simulink model "modelo_2"  (R2020a)
settings: Solver=VariableStepAuto  StartTime=0.0  StopTime=180  RelTol=1e-3
values from neighbouring files (symbols this model uses):
  Pnom = 2e6    (= 2000000)    [Parametros.m]
  Pnom1 = 2e6    (= 2000000)    [Parametros.m]
libraries: powerlib x7, re_lib x2, powerlib_meascontrol x1
settings Model: Creator=octad  LastModifiedBy=octad

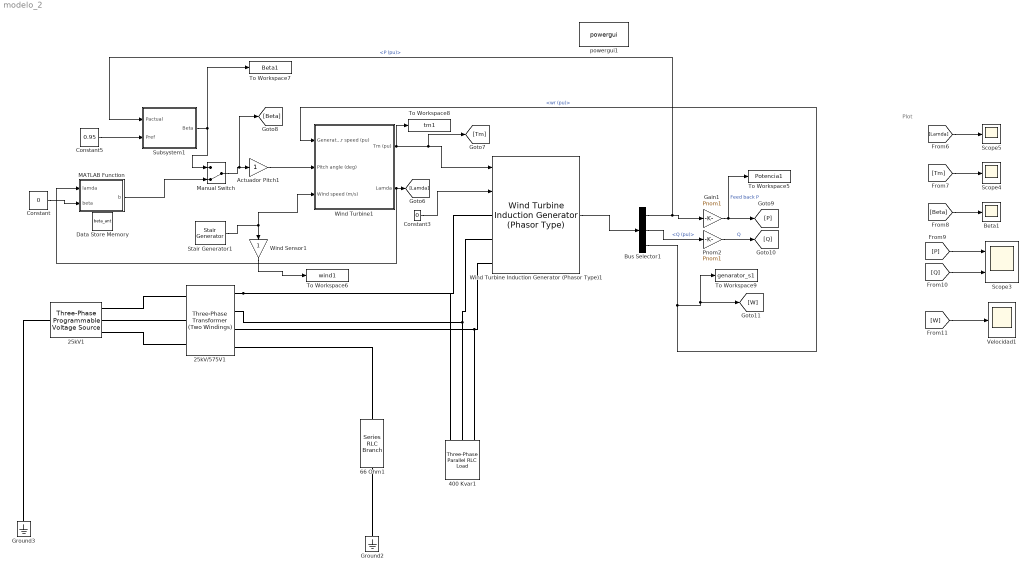
== system modelo_2 ==
  note: Plot
  25kV/575V1 : powerlib/Elements/Three-Phase Transformer (Two Windings)  Winding1Connection=Yg  Winding2Connection=Yn  CoreType=Three single-phase transformers  SetSaturation=off  Hysteresis=off  DataFile='hysteresis'  SetInitialFlux=off  Measurements=None  UNITS=pu  NominalPower=[ 4e6 , 60 ]  Winding1=[ 25e3 , 0.025/30 , 0.025]  Winding2=[575 , 0.025/30 , 0.025 ]  Rm=500  Lm=inf  L0=0.5  Saturation=[ 0,0 ; 0.0024,1.2 ; 1.0,1.52 ]  InitialFluxes=[ 0.8 , -0.8 , 0.7 ]  BreakLoop=off  DiscreteSolver=Trapezoidal iterative  DataType=off  TransfoNumber=1
  25kV1 : powerlib/Electrical Sources/Three-Phase Programmable Voltage Source  PositiveSequence="[25000  0 60]"  VariationEntity=None  VariationType=Table of time-amplitude pairs  VariationTypeAlt=Step  VariationStep=0.5  VariationRate=10  VariationMagnitude=0.3  VariationFrequency=2  VariationTiming=[1 2]  VariationPhaseA=off  Amplitudes=[1 0.8 1.2 1.0]  TimeValues=[0 0.1 0.15 0.2]  HarmonicGeneration=off  HarmonicA=[3 0.2 -25 0]  HarmonicB=[2 0.15 35 2]  Timing="[0.05  3]"  BusType=swing  Pref=0  Qref=0  Qmin=-inf  Qmax=inf
  400 Kvar1 : powerlib/Elements/Three-Phase Parallel RLC Load  LConnTagsString=A|B|C  Configuration=Delta  NominalVoltage=575  Vabc=[1e3 1e3 1e3]  Vabcp=[1e3 1e3 1e3]  NominalFrequency=60  UnbalancedPower=off  ActivePower=0  InductivePower=0  CapacitivePower=400e3  Pabc=[10e3 9e3 11e3]  QLabc=[100 90 110]  QCabc=[100 90 110]  Pabcp=[10e3 9e3 11e3]  QLabcp=[100 90 110]  QCabcp=[100 90 110]  Measurements=None  LoadType=constant Z
  66 Ohm1 : powerlib/Elements/Series RLC Branch  LConnTagsString=__new0  RConnTagsString=__new0  BranchType=R  Resistance=66  Inductance=1e-3  SetiL0=off  InitialCurrent=0  Capacitance=1e-6  Setx0=off  InitialVoltage=0  Measurements=None
  Actuador Pitch1 : Gain
  Beta1 : Scope
  Bus Selector1 : BusSelector  OutputSignals=P (pu),Q (pu),wr (pu)
  Constant : Constant  Value=0
  Constant3 : Constant  Value=0
  Constant5 : Constant  Value=0.95
  Data Store Memory : DataStoreMemory  DataStoreName=beta_ant  ReadBeforeWriteMsg=warning  WriteAfterWriteMsg=warning  WriteAfterReadMsg=warning  ShowAdditionalParam=off  OutDataTypeStr=double
  Gain1 : Gain  Gain=Pnom1
  Ground2 : powerlib/Elements/Ground  LConnTagsString=a
  Ground3 : powerlib/Elements/Ground  LConnTagsString=a
  MATLAB Function : MATLAB Function  TreatAsAtomicUnit=on
  Manual Switch : ManualSwitch  CurrentSetting=0
  Pnom2 : Gain  Gain=Pnom1
  Scope3 : Scope  NumInputPorts=2
  Scope4 : Scope
  Scope5 : Scope
  Stair Generator1 : powerlib_meascontrol/Pulse & Signal Generators/Stair Generator  t=[0, 10, 20, 30, 40, 60,70,90]  e=[3, 7, 11, 13, 18, 13,11,12]  Ts=0
  Subsystem1 : Subsystem
  To Workspace5 : ToWorkspace  VariableName=Potencia1  SaveFormat=Timeseries  SampleTime=-1
  To Workspace6 : ToWorkspace  VariableName=wind1  SaveFormat=Timeseries  SampleTime=-1
  To Workspace7 : ToWorkspace  VariableName=Beta1  SaveFormat=Timeseries  SampleTime=-1
  To Workspace8 : ToWorkspace  VariableName=tm1  SaveFormat=Timeseries  SampleTime=-1
  To Workspace9 : ToWorkspace  VariableName=genarator_s1  SaveFormat=Timeseries  SampleTime=-1
  Velocidad1 : Scope
  Wind Sensor1 : Gain
  Wind Turbine Induction Generator (Phasor Type)1 : re_lib/Wind Generation/Wind Turbine Induction Generator (Phasor Type)  ExternalTm=on  nom=[Pnom1/0.9, 575, 60]  sta=[ 0.004843, 0.1248]  rot=[ 0.004377, 0.1791]  Lm=6.77  mec=[5.04, 0.01, 3]  init="[ -0.01,0,   0,0,0,   0,0,0 ]"  pitch_angle=0  Pmec=1.5e6  wind_base=12  speed_nom=1  P_wind_base=1  K_pitch_gain=[5 25]  pitch_max=45  pitch_rate=2
      settings: SourceProductBaseCode=PS
  Wind Turbine1 : Subsystem  AncestorBlock=re_lib/Wind Generation/Wind Turbine  DialogController=POWERSYS.PowerSysDialog  mask(Wind Turbine){Pnom=Pnom, Pelec_base=Pnom1/0.9, wind_base=12, P_wind_base=0.5, speed_nom=1, pitch_angle=0, c1_c6=[0.51763          116          0.4            5           21     0.006795], cp_nom=0.48, lambda_nom=8.1}
      mask prompts: Pnom "Nominal mechanical output power (W):"; Pelec_base "Base power of the electrical generator (VA):"; wind_base "Base wind speed (m/s):"; P_wind_base "Maximum power at base wind speed (pu of nominal mechanical power):"; speed_nom "Base rotational speed (p.u. of base generator speed):"; pitch_angle "Pitch angle beta to display wind-turbine power characteristics (beta >=0)  (deg):"
      mask help:
      | This block implements a variable pitch wind turbine model. The performance coefficient Cp of the turbine is the mechanical output power of the turbine divided by wind power and a function of wind speed, rotational speed, and pitch angle (beta). Cp reaches its maximum value at zero beta. Select the wind-turbine power characteristics display to plot the turbine characteristics at the specified pitch angle.
      |
      | The first input is the generator speed in per unit of the generator base speed. For a synchronous or asynchronous generator, the base speed is the synchronous speed. For a permanent-magnet generator, the base speed is defined as the speed producing nominal voltage at  no load. The second input is the blade pitch angle (beta) in degrees. The third input is the wind speed in m/s.
      |
      | The output is the torque applied to the generator shaft in per unit of the generator ratings.
      |
      | The turbine inertia must be added to the generator inertia.
      mask init:
      | c1=c1_c6(1);c2=c1_c6(2);c3=c1_c6(3);c4=c1_c6(4);c5=c1_c6(5);c6=c1_c6(6);
      | 
      | if Pnom<=0
      |     error(message('physmod:powersys:common:GreaterThan',getfullname(gcbh),'Nominal mechanical output power',0));
      | end
      | if Pelec_base<=0
      |     error(message('physmod:powersys:common:GreaterThan',getfullname(gcbh),'Base power of the electrical generator',0));
      | end
      | if wind_base<=0
      |     error(message('physmod:powersys:common:GreaterThan',getfullname(gcbh),'Base wind speed (m/s)',0));
      | end
      | if P_wind_base<=0
      |     error(message('physmod:powersys:common:GreaterThan',getfullname(gcbh),'Maximum power at base wind speed',0));
      | end
      | power_initmask();
      settings: OpenFcn=sps_rtmsupport('OpenFcn',gcbh)
      mask Help: helpview(psbhelp);
      mask DialogControl DisplayTurbChar Prompt: Display wind turbine power characteristics
      mask DialogControl DisplayTurbChar Callback: WindTurbinePlot(gcb)
      mask Display: disp('');
  powergui1 : powerlib/powergui  Priority=1  SimulationMode=Phasor  SampleTime=50e-6  frequency=60  Iterations=50  frequencyindice=60  Pbase=100e6  ErrMax=1e-4  UnitsV=kV  UnitsW=MW  buscounter=0  FunctionMessages=off  echomessages=off  EnableUseOfTLC=off  CurrentSourceSwitches=off  DisableSnubberDevices=off  DisableRonSwitches=off  DisableVfSwitches=off  DisplayEquations=off  AutomaticDiscreteSolvers=off  SolverType=Tustin/Backward Euler (TBE)  Interpol=off  ExternalGateDelay=off  methode=off  Ts=100  x0status=blocks  SPID=on  SwTol=0  HookPort=off  NonlinearTolerance=1e-4  nMaxIteration=100  ContinueOnMaxIteration=off  RestoreLinks=warning  ResistiveCurrentMeasurement=off  Frange=[0:2:500]  Ylog=off  Xlog=on  ShowGrid=off  save=off  variable=ZData  structure=0  ZoomFFT=off  StartTime=0.0  cycles=1  DisplayStyle=1  fundamental=60  FreqAxis=off  MaxFrequency=1000  frequencyindicesteady=1  RmsSteady=1  display=off
  wires:
  Actuador Pitch1/1 -> Wind Turbine1/2(Pitch angle (deg))
  Wind Sensor1/1 -> To Workspace6/1
  Wind Turbine1/2(Lamda) -> MATLAB Function/1(lamda), [Lamda]
  [P] -> Scope3/1
  Constant5/1 -> Subsystem1/2(Pref)
  Constant3/1 -> Wind Turbine Induction Generator (Phasor Type)1/2
  Wind Turbine Induction Generator (Phasor Type)1/1 -> Bus Selector1/1
  Bus Selector1/3 -> [W], To Workspace9/1, Wind Turbine1/1(Generator speed (pu))  "<wr (pu)>"
  Gain1/1 -> [P], To Workspace5/1  "Feed back P"
  Subsystem1/1(Beta) -> Manual Switch/1, To Workspace7/1
  Wind Turbine1/1(Tm (pu)) -> [Tm], Wind Turbine Induction Generator (Phasor Type)1/1, To Workspace8/1
  Bus Selector1/1 -> Subsystem1/1(Pactual), Gain1/1  "<P (pu)>"
  [W] -> Velocidad1/1
  Pnom2/1 -> [Q]  "Q"
  [Tm] -> Scope4/1
  Bus Selector1/2 -> Pnom2/1  "<Q (pu)>"
  [Beta] -> Beta1/1
  [Lamda] -> Scope5/1
  Stair Generator1/1 -> Wind Turbine1/3(Wind speed (m/s)), Wind Sensor1/1
  [Q] -> Scope3/2
  MATLAB Function/1(b) -> Manual Switch/2
  Manual Switch/1 -> [Beta], Actuador Pitch1/1
  Constant/1 -> MATLAB Function/2(beta)
  connections:
  25kV/575V1/RConn3 -- 400 Kvar1/LConn3 -- Wind Turbine Induction Generator (Phasor Type)1/LConn3
  25kV/575V1/RConn1 -- 400 Kvar1/LConn1 -- Wind Turbine Induction Generator (Phasor Type)1/LConn1
  25kV/575V1/RConn2 -- Wind Turbine Induction Generator (Phasor Type)1/LConn2 -- 400 Kvar1/LConn2
  25kV/575V1/RConn4 -- 66 Ohm1/LConn1
  Ground3/LConn1 -- 25kV1/LConn1
  25kV1/RConn3 -- 25kV/575V1/LConn3
  25kV1/RConn2 -- 25kV/575V1/LConn2
  25kV1/RConn1 -- 25kV/575V1/LConn1
  Ground2/LConn1 -- 66 Ohm1/RConn1

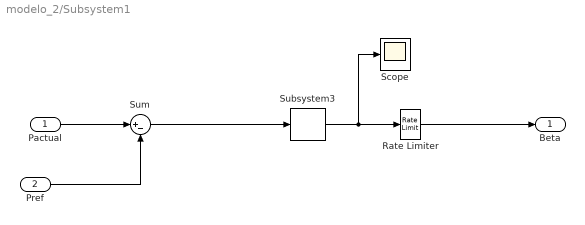
== system modelo_2/Subsystem1 ==
  Pactual : Inport
  Pref : Inport  Port=2
  "Rate Limiter   " : RateLimiter  RisingSlewLimit=2  FallingSlewLimit=-2
  Scope : Scope
  Subsystem3 : re_lib/Wind Generation/Wind Turbine Induction Generator (Phasor Type)/Subsystem3  Kp=5  Ki=25  Limits=[45 0]  Init=0
      settings: SourceProductBaseCode=PS
  Sum : Sum  Inputs=|+-
  Beta : Outport
  wires:
  Pref/1 -> Sum/2
  Subsystem3/1 -> Scope/1, "Rate Limiter   "/1
  "Rate Limiter   "/1 -> Beta/1
  Pactual/1 -> Sum/1
  Sum/1 -> Subsystem3/1

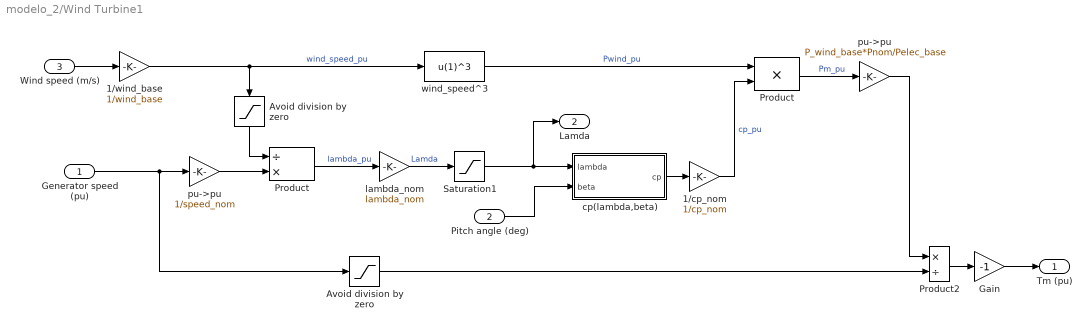
== system modelo_2/Wind Turbine1 ==
  Generator speed (pu) : Inport
  Pitch angle (deg) : Inport  Port=2
  Wind speed (m/s) : Inport  Port=3
  1/cp_nom : Gain  Gain=1/cp_nom  SaturateOnIntegerOverflow=on  OutDataTypeStr=Inherit: Same as input  ParamDataTypeStr=Inherit: Same as input
  1/wind_base : Gain  Gain=1/wind_base  SaturateOnIntegerOverflow=on  OutDataTypeStr=Inherit: Same as input  ParamDataTypeStr=Inherit: Same as input
  Avoid division by zero : Saturate  UpperLimit=1e6  LowerLimit=1e-6
  "Avoid division by zero " : Saturate  UpperLimit=inf  LowerLimit=1e-6
  Gain : Gain  Gain=-1  SaturateOnIntegerOverflow=on  OutDataTypeStr=Inherit: Same as input  ParamDataTypeStr=Inherit: Same as input
  Product : Product  Inputs=/*  SaturateOnIntegerOverflow=on  OutDataTypeStr=Inherit: Same as first input
  "Product " : Product  SaturateOnIntegerOverflow=on  OutDataTypeStr=Inherit: Same as first input
  Product2 : Product  Inputs=*/  InputSameDT=on  SaturateOnIntegerOverflow=on  OutDataTypeStr=Inherit: Same as first input
  Saturation1 : Saturate  UpperLimit=inf  LowerLimit=1e-6
  cp(lambda,beta) : Subsystem
  lambda_nom : Gain  Gain=lambda_nom  SaturateOnIntegerOverflow=on  OutDataTypeStr=Inherit: Same as input  ParamDataTypeStr=Inherit: Same as input
  pu->pu : Gain  Gain=P_wind_base*Pnom/Pelec_base  SaturateOnIntegerOverflow=on  OutDataTypeStr=Inherit: Same as input  ParamDataTypeStr=Inherit: Same as input
  "pu->pu " : Gain  Gain=1/speed_nom  SaturateOnIntegerOverflow=on  OutDataTypeStr=Inherit: Same as input  ParamDataTypeStr=Inherit: Same as input
  wind_speed^3 : Fcn  Expr=u(1)^3
  Tm (pu) : Outport  VectorParamsAs1DForOutWhenUnconnected=off
  Lamda : Outport  Port=2
  wires:
  Pitch angle (deg)/1 -> cp(lambda,beta)/2(beta)
  pu->pu/1 -> Product2/1
  cp(lambda,beta)/1(cp) -> 1/cp_nom/1
  wind_speed^3/1 -> "Product "/1  "Pwind_pu"
  Product2/1 -> Gain/1
  Avoid division by zero/1 -> Product2/2
  Wind speed (m/s)/1 -> 1/wind_base/1
  Gain/1 -> Tm (pu)/1
  Generator speed (pu)/1 -> Avoid division by zero/1, "pu->pu "/1
  "Product "/1 -> pu->pu/1  "Pm_pu"
  lambda_nom/1 -> Saturation1/1  "Lamda"
  1/cp_nom/1 -> "Product "/2  "cp_pu"
  Saturation1/1 -> cp(lambda,beta)/1(lambda), Lamda/1
  Product/1 -> lambda_nom/1  "lambda_pu"
  1/wind_base/1 -> wind_speed^3/1, "Avoid division by zero "/1  "wind_speed_pu"
  "Avoid division by zero "/1 -> Product/1
  "pu->pu "/1 -> Product/2

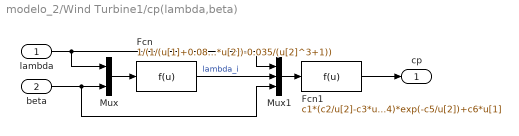
== system modelo_2/Wind Turbine1/cp(lambda,beta) ==
  lambda : Inport
  beta : Inport  Port=2
  Fcn : Fcn  Expr=1/(1/(u[1]+0.08*u[2])-0.035/(u[2]^3+1))
  Fcn1 : Fcn  Expr=c1*(c2/u[2]-c3*u[3]-c4)*exp(-c5/u[2])+c6*u[1]
  Mux : Mux  Inputs=2
  Mux1 : Mux  Inputs=3
  cp : Outport  VectorParamsAs1DForOutWhenUnconnected=off
  wires:
  Fcn/1 -> Mux1/2  "lambda_i"
  Fcn1/1 -> cp/1
  lambda/1 -> Mux1/1, Mux/1
  Mux1/1 -> Fcn1/1
  beta/1 -> Mux1/3, Mux/2
  Mux/1 -> Fcn/1

== matlab function modelo_2/MATLAB Function ==
  settings: updateMethod=DISCRETE
  data: lamda input; b output; beta input; beta_ant data_store_memory
function b = fcn(lamda, beta)
global beta_ant;

b= s_annealing(lamda, beta);
beta_ant=b;
end
